simulink model "Transfert_Function"  (R2024a)
settings: Solver=VariableStepAuto  StartTime=0.0  StopTime=10  RelTol=1e-3
settings Model: Creator=yoanp  LastModifiedBy=yoanp

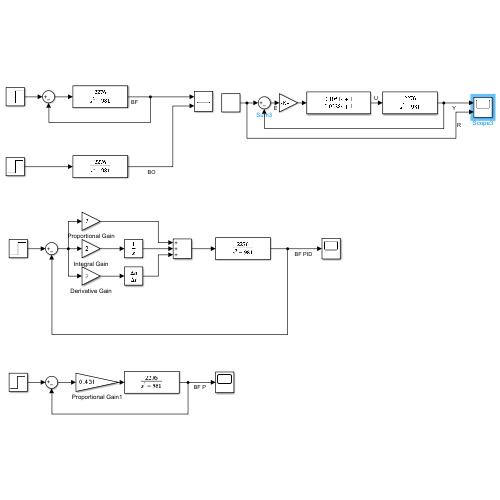
[thumbnail: Simulink's stored preview of the top-level diagram]
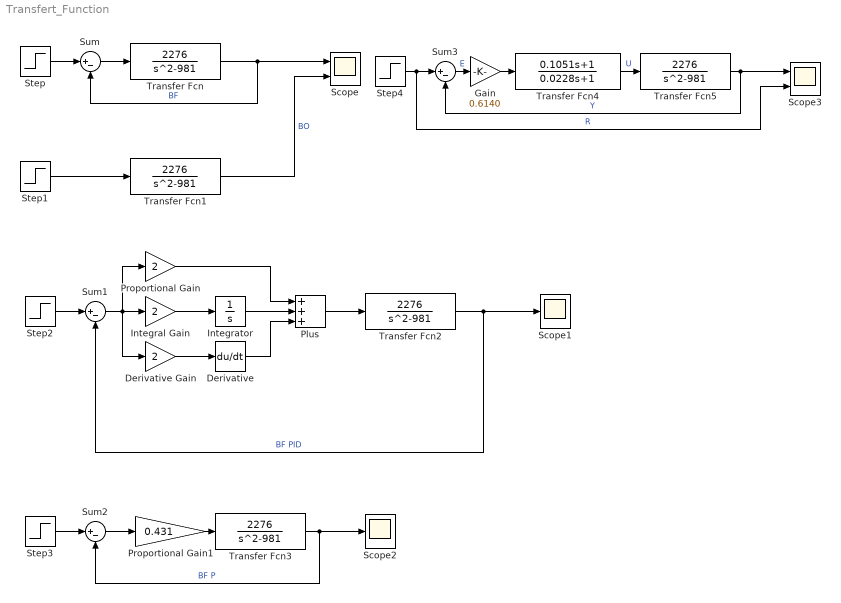
== system Transfert_Function ==
  Derivative : Derivative
  Derivative Gain : Gain  Gain=2
  Gain : Gain  Gain=0.6140
  Integral Gain : Gain  Gain=2
  Integrator : Integrator
  Plus : Sum  Inputs=+++
  Proportional Gain : Gain  Gain=2
  Proportional Gain1 : Gain  Gain=0.431
  Scope : Scope  NumInputPorts=2
  Scope1 : Scope
  Scope2 : Scope
  Scope3 : Scope  NumInputPorts=2
  Step{,1..4} (5 alike) : Step  SampleTime=0
  Sum{,1..3} (4 alike) : Sum  Inputs=|+-
  Transfer Fcn{,1..3,5} (5 alike) : TransferFcn  Numerator=[2276]  Denominator=[1 0 -981]
  Transfer Fcn4 : TransferFcn  Numerator=[0.1051 1]  Denominator=[0.0228 1]
  wires:
  Transfer Fcn/1 -> Scope/1, Sum/2  "BF"
  Step/1 -> Sum/1
  Sum/1 -> Transfer Fcn/1
  Step1/1 -> Transfer Fcn1/1
  Transfer Fcn1/1 -> Scope/2  "BO"
  Transfer Fcn2/1 -> Scope1/1, Sum1/2  "BF PID"
  Step2/1 -> Sum1/1
  Sum1/1 -> Derivative Gain/1, Proportional Gain/1, Integral Gain/1
  Derivative Gain/1 -> Derivative/1
  Plus/1 -> Transfer Fcn2/1
  Derivative/1 -> Plus/3
  Integrator/1 -> Plus/2
  Proportional Gain/1 -> Plus/1
  Integral Gain/1 -> Integrator/1
  Step3/1 -> Sum2/1
  Transfer Fcn3/1 -> Sum2/2, Scope2/1  "BF P"
  Sum2/1 -> Proportional Gain1/1
  Proportional Gain1/1 -> Transfer Fcn3/1
  Transfer Fcn5/1 -> Scope3/1, Sum3/2  "Y"
  Step4/1 -> Scope3/2, Sum3/1  "R"
  Transfer Fcn4/1 -> Transfer Fcn5/1  "U"
  Sum3/1 -> Gain/1  "E"
  Gain/1 -> Transfer Fcn4/1
